simulink model "Signal_sampling_and_interpolation"  (R2016b)
settings: Solver=VariableStepAuto  StartTime=0.0  StopTime=10.0  RelTol=1e-3
libraries: dsparch4 x2
settings Model: Creator=yang guo  LastModifiedBy=yang guo

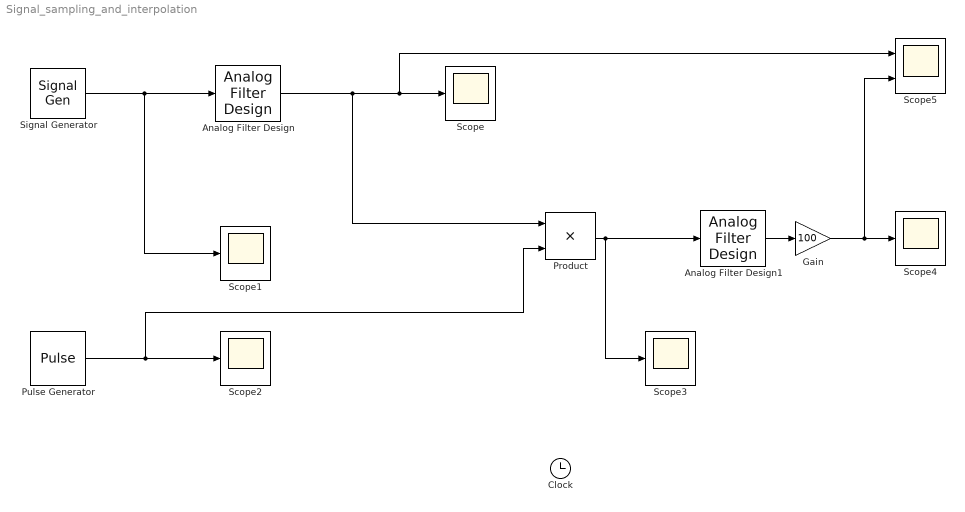
== system Signal_sampling_and_interpolation ==
  Analog Filter Design : dsparch4/Analog Filter Design  method=Butterworth  filttype=Lowpass  N=8  Wlo=20*pi  Whi=80  Rp=2  Rs=40
  Analog Filter Design1 : dsparch4/Analog Filter Design  method=Butterworth  filttype=Lowpass  N=8  Wlo=62*pi  Whi=20*pi  Rp=2  Rs=40
  Clock : Clock
  Gain : Gain  Gain=100
  Product : Product
  Pulse Generator : DiscretePulseGenerator  PulseType=Time based  Period=0.01
  Scope{,1..4} (5 alike) : Scope
  Scope5 : Scope  NumInputPorts=2
  Signal Generator : SignalGenerator  Amplitude=3  Frequency=6
  wires:
  Signal Generator/1 -> Scope1/1, Analog Filter Design/1
  Analog Filter Design/1 -> Product/1, Scope5/1, Scope/1
  Pulse Generator/1 -> Product/2, Scope2/1
  Product/1 -> Scope3/1, Analog Filter Design1/1
  Gain/1 -> Scope5/2, Scope4/1
  Analog Filter Design1/1 -> Gain/1
